simulink model "si3_state_port"  (R2017a)
settings: Solver=VariableStepAuto  StartTime=0.0  StopTime=6  MaxStep=0.2  RelTol=1e-3
settings Model: Creator=Bob  LastModifiedBy=Bob

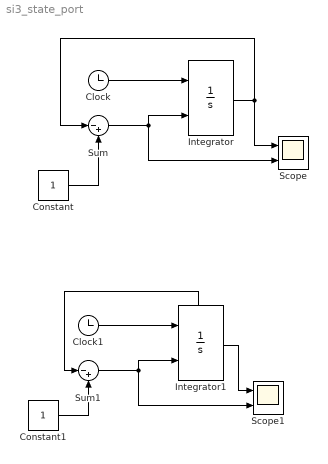
== system si3_state_port ==
  Clock : Clock
  Clock1 : Clock
  Constant : Constant
  Constant1 : Constant
  Integrator : Integrator  ExternalReset=falling
  Integrator1 : Integrator  ExternalReset=falling  ShowStatePort=on
  Scope : Scope  NumInputPorts=2
  Scope1 : Scope  NumInputPorts=2
  Sum : Sum  Inputs=|-+
  Sum1 : Sum  Inputs=|-+
  wires:
  Clock/1 -> Integrator/1
  Sum/1 -> Scope/2, Integrator/2
  Constant/1 -> Sum/2
  Constant1/1 -> Sum1/2
  Clock1/1 -> Integrator1/1
  Integrator1/1 -> Scope1/1
  Sum1/1 -> Scope1/2, Integrator1/2
  Integrator1/State -> Sum1/1
  Integrator/1 -> Scope/1, Sum/1
